simulink model "basic_cosimulation_c_1_sm_master"  (R2021b)
settings: Solver=ode4  StartTime=0.0  StopTime=inf  FixedStep=5e-05  RelTol=1e-3  EnableMultiTasking=on
PostLoadFcn:
  | %
  | % Script for validation of swtiching model design with it's respective
  | % average model.
  | %
  | % Here it is presented the design of the inverter to the 6 kW Fuel Cell
  | % model.
  | 
  | %%% Initialization %%%
  | 
  | 
  | % ------------------------------------- %
  | % ---------- Inverter Design ---------- %
  | % ------------------------------------- %
  | 
  | %%%% Nominal Parameters %%%%
  | 
  | Pnom = 50e3;                                        % Nominal Power
  | Vdc = 400;                                          % DC Voltage - Boost
  | m = 0.6;                                            % Modulation Index
  | Vnom_peak = m*Vdc/2;                                % Peak Voltage
  | Vnom_rms = Vnom_peak/sqrt(2);                       % Rms Voltage
  | FP_min = 0.9;                                       % For Reactive Power
  |                                                     % Compensation
  | Snom = Pnom/FP_min;                                 % Apparent Power
  | Irms = Pnom/(sqrt(3)*Vnom_rms);                     % Rms Curren
  | Inom_peak = Irms*sqrt(2);                           % Peak Current
  | Zbase = Vnom_peak/Inom_peak;                        % Base Impedance
  | f = 60;                                             % Nominal Frequency
  | wnom = 2*pi*60;                                     % Angular Frequency
  | 
  | % ------------------------- %
  | % Inverter LC Filter Design %
  | % ------------------------- %
  | 
  | fsw_inv = 96*60;                                    % Switching Frequency must be a multiple of the nominal frequency
  |                                                      % for proper operation of the Artemis Block
  | ripple_inv = 0.03;
  | L_inv = ((Vdc/2)-Vnom_peak)*(1/fsw_inv)/(ripple_inv*Inom_peak);
  | 
  | % - Capacitor
  | fres = 420;                                         % Filters Ressonant Frequency
  | 
  | Cf = 1/(4*L_inv*(pi^2)*(fres^2));                % Filter Capacitor
  | Rf = 1/(wnom*Cf*50);                                % Damping Resistor
  | 
  | % --- Sample Time --- %
  | 
  | Tsw = 0.00050;
  | Ts = Tsw/10;
  | 
  | % ---------------------- %
  | % Current Control Design %
  | % ---------------------- %
  | 
  | Ron = 0.001;                                        % IGBT Resistance
  | tau_i = 1e-3;                                       % Responde Time
  | kp_current = L_inv/tau_i;                           % PI Proportional Gain
  | ki_current = (Ron)/tau_i;                           % PI Integral Gain
  | 
  | decouple = (wnom*L_inv);                            % Decoupling Gain
InitFcn:
  | %
  | % Script for validation of swtiching model design with it's respective
  | % average model.
  | %
  | % Here it is presented the design of the inverter to the 6 kW Fuel Cell
  | % model.
  | 
  | %%% Initialization %%%
  | 
  | 
  | % ------------------------------------- %
  | % ---------- Inverter Design ---------- %
  | % ------------------------------------- %
  | 
  | %%%% Nominal Parameters %%%%
  | 
  | Pnom = 50e3;                                        % Nominal Power
  | Vdc = 400;                                          % DC Voltage - Boost
  | m = 0.6;                                            % Modulation Index
  | Vnom_peak = m*Vdc/2;                                % Peak Voltage
  | Vnom_rms = Vnom_peak/sqrt(2);                       % Rms Voltage
  | FP_min = 0.9;                                       % For Reactive Power
  |                                                     % Compensation
  | Snom = Pnom/FP_min;                                 % Apparent Power
  | Irms = Pnom/(sqrt(3)*Vnom_rms);                     % Rms Curren
  | Inom_peak = Irms*sqrt(2);                           % Peak Current
  | Zbase = Vnom_peak/Inom_peak;                        % Base Impedance
  | f = 60;                                             % Nominal Frequency
  | wnom = 2*pi*60;                                     % Angular Frequency
  | 
  | % ------------------------- %
  | % Inverter LC Filter Design %
  | % ------------------------- %
  | 
  | fsw_inv = 96*60;                                    % Switching Frequency must be a multiple of the nominal frequency
  |                                                      % for proper operation of the Artemis Block
  | ripple_inv = 0.03;
  | L_inv = ((Vdc/2)-Vnom_peak)*(1/fsw_inv)/(ripple_inv*Inom_peak);
  | 
  | % - Capacitor
  | fres = 420;                                         % Filters Ressonant Frequency
  | 
  | Cf = 1/(4*L_inv*(pi^2)*(fres^2));                % Filter Capacitor
  | Rf = 1/(wnom*Cf*50);                                % Damping Resistor
  | 
  | % --- Sample Time --- %
  | 
  | Tsw = 0.00050;
  | Ts = Tsw/10;
  | 
  | % ---------------------- %
  | % Current Control Design %
  | % ---------------------- %
  | 
  | Ron = 0.001;                                        % IGBT Resistance
  | tau_i = 1e-3;                                       % Responde Time
  | kp_current = L_inv/tau_i;                           % PI Proportional Gain
  | ki_current = (Ron)/tau_i;                           % PI Integral Gain
  | 
  | decouple = (wnom*L_inv);                            % Decoupling Gain
undefined symbols (not defined in the file or in its folder): D1, Delta, DiscIntNeverNeededParam, IP, j, ph, sps, UDP
libraries: powerlib x85, rtlab x16, spsCurrentMeasurementLib x11, powerlib_meascontrol x10, simulink x8, rteventslib x8, ssn_inverter_model x4, eePowerMeasurement x4, spsThreePhaseSeriesRLCBranchLib x4, spsVoltageMeasurementLib x4, opal_lib x3, spsUniversalBridgeLib x3
(part 2 of 5)

== system basic_cosimulation_c_1_sm_master/SM_Master/Circuit_ITM_Source_DP_AW ==
  Data_In : Inport
  AC Voltage Source : powerlib/Electrical Sources/AC Voltage Source  Commented=on  Amplitude=100  Phase=0  Frequency=60  SampleTime=0  Measurements=None  BusType=swing  Pref=10e3  Qref=0  Qmin=-inf  Qmax=+inf
  Amplitude : Step  Time=3  Before=220*sqrt(2/3)  After=220*sqrt(2/3)*0.8  SampleTime=Ts
  "Amplitude1 " : Step  Time=4  After=-220*sqrt(2/3)*0.2  SampleTime=Ts
  Constant : Constant  Commented=on  Value=5/60  SampleTime=Ts
  "Controllable Voltage Source " : Subsystem
  Controlled Current Source : powerlib/Electrical Sources/Controlled Current Source  Commented=on  Initialize=on  Source_Type=AC  Amplitude=0  Phase=0  Frequency=0  Measurements=None
  DP - > EMT : Subsystem
  DP --> EMT : Subsystem  Commented=on
  Demux1 : Demux  Outputs=3
  Digital Clock : DigitalClock  Commented=on  SampleTime=Ts
  Dynamic Phasor coeficientes extraction : Subsystem
  Dynamic Phasor coeficients extraction : Subsystem  Commented=on
  Freq : Step  Time=2.8  After=-2  SampleTime=Ts
  Freq Ref : Step  Time=2  Before=60  After=58  SampleTime=Ts
  GreaterThan : RelationalOperator  Commented=on  Operator=>  OutDataTypeStr=boolean  RndMeth=Simplest
  Ground1 : powerlib/Elements/Ground  Commented=on  LConnTagsString=a
  Mux : Mux  Inputs=3
  Mux1 : Mux  Inputs=3
  Phase Ref : Constant  Value=0  SampleTime=Ts
  Series RLC Branch : powerlib/Elements/Series RLC Branch  Commented=on  LConnTagsString=__new0  RConnTagsString=__new0  BranchType=R  Resistance=0.5  Inductance=1e-3  SetiL0=off  InitialCurrent=0  Capacitance=1e-6  Setx0=off  InitialVoltage=0  Measurements=None
  Subsystem : Subsystem  Commented=on
  Sum : Sum  Inputs=-+|
  Sum1 : Sum  Inputs=|+-
  Three-Phase Series RLC Branch1 : powerlib/Elements/Three-Phase Series RLC Branch  LConnTagsString=A|B|C  RConnTagsString=A|B|C  BranchType=R  Resistance=2  Inductance=1e-3  Capacitance=1e-6  Measurements=None
  Three-Phase V-I Measurement : powerlib/Measurements/Three-Phase V-I Measurement  VoltageMeasurement=phase-to-ground  SetLabelV=off  LabelV=Vabc  Vpu=off  VpuLL=off  CurrentMeasurement=yes  SetLabelI=off  LabelI=Iabc  Ipu=off  Pbase=100e6  Vbase=25e3  OutputType=Complex  PhasorSimulation=off  PSBequivalent=0
  Three-Phase Controlled Y-Connected Current Source : Subsystem
      settings: PortSchema="{\"entries\":[{\"content\":{\"sides\":[{\"content\":{\"connectorIds\":[\"LConn1\",\"LConn2\",\"LConn3\"]},\"type\":\"ConnectorPlacement.EquallySpacedRectSide\",\"uuid\":\"a8a67328-a09d-4495-b33c-aaf3ca0795cb\"},{\"content\":{\"connectorIds\":[\"In1\",\"In2\",\"In3\"],\"side\":\"RIGHT\"},\"type\":\"ConnectorPlacement.EquallySpacedRectSide\",\"uuid\":\"ca8d97e2-0dea-49aa-8cb7-235b4eace1f8\"},{\"content\":{\"connectorIds\":[],\"side\":\"TOP\"},\"type\":\"ConnectorPlacement.EquallySpacedRectSide\",\"uuid\":\"ab6aade9-1d27-4135-8ce1-c4358d4ecc87\"}]},\"type\":\"ConnectorPlacement.EquallySpacedConnector\",\"uuid\":\"205b5c38-55ea-4d68-a706-de660c21807c\"}],\"packageUris\":[\"http://schema.mathworks.com/mf0/Connector/19700101\"],\"version\":\"1.0\"}"
  Voltage Measurement : powerlib/Measurements/Voltage Measurement  Commented=on  PhasorSimulation=off  OutputType=Complex  PSBequivalent=0
  Vabc_Phasor_out : Outport
  I_injected : Outport  Port=2
  wires:
  DP --> EMT/1(I_injected) -> Controlled Current Source/1
  Voltage Measurement/1 -> Dynamic Phasor coeficients extraction/1(EMT Signal)
  Dynamic Phasor coeficients extraction/1(Mag) -> ?
  Dynamic Phasor coeficients extraction/2(Phase) -> ?
  Data_In/1 -> Demux1/1
  Three-Phase V-I Measurement/1 -> Dynamic Phasor coeficientes extraction/1(EMT_Signal)
  Dynamic Phasor coeficientes extraction/3(Phasor_C) -> Mux/3
  Dynamic Phasor coeficientes extraction/2(Phasor_B) -> Mux/2
  Dynamic Phasor coeficientes extraction/1(Phasor_A) -> Mux/1
  Mux/1 -> Vabc_Phasor_out/1
  Demux1/1 -> DP - > EMT/1(Phasor_A)
  Demux1/2 -> DP - > EMT/2(Phasor_B)
  Demux1/3 -> DP - > EMT/3(Phasor_C)
  DP - > EMT/2(Sinal_B) -> Mux1/2, Three-Phase Controlled Y-Connected Current Source/2(Ib)
  DP - > EMT/1(Sinal_A) -> Mux1/1, Three-Phase Controlled Y-Connected Current Source/1(Ia)
  DP - > EMT/3(Sinal_C) -> Mux1/3, Three-Phase Controlled Y-Connected Current Source/3(Ic)
  Mux1/1 -> I_injected/1
  Digital Clock/1 -> GreaterThan/1
  Constant/1 -> GreaterThan/2
  GreaterThan/1 -> ?
  Freq/1 -> Sum1/2
  Amplitude/1 -> Sum/2
  Sum/1 -> "Controllable Voltage Source "/1(Amplitude [V])
  Freq Ref/1 -> Sum1/1
  "Amplitude1 "/1 -> Sum/1
  Sum1/1 -> "Controllable Voltage Source "/3(Frequency [Hz])
  Phase Ref/1 -> "Controllable Voltage Source "/2(Phase [Deg])
  connections:
  AC Voltage Source/RConn1 -- Series RLC Branch/LConn1
  AC Voltage Source/LConn1 -- Controlled Current Source/RConn1 -- Voltage Measurement/LConn2 -- Ground1/LConn1
  Series RLC Branch/RConn1 -- Voltage Measurement/LConn1 -- Controlled Current Source/LConn1
  Three-Phase Series RLC Branch1/RConn2 -- Three-Phase V-I Measurement/LConn2
  Three-Phase V-I Measurement/LConn3 -- Three-Phase Series RLC Branch1/RConn3
  Three-Phase V-I Measurement/LConn1 -- Three-Phase Series RLC Branch1/RConn1
  Three-Phase Controlled Y-Connected Current Source/LConn1 -- Three-Phase V-I Measurement/RConn1
  Three-Phase V-I Measurement/RConn2 -- Three-Phase Controlled Y-Connected Current Source/LConn2
  Three-Phase V-I Measurement/RConn3 -- Three-Phase Controlled Y-Connected Current Source/LConn3
  "Controllable Voltage Source "/RConn1 -- Three-Phase Series RLC Branch1/LConn1
  Three-Phase Series RLC Branch1/LConn2 -- "Controllable Voltage Source "/RConn2
  Three-Phase Series RLC Branch1/LConn3 -- "Controllable Voltage Source "/RConn3

== system basic_cosimulation_c_1_sm_master/SM_Master/Circuit_ITM_Source_DP_SFA ==
  Data_In : Inport
  AC Voltage Source : powerlib/Electrical Sources/AC Voltage Source  Commented=on  Amplitude=100  Phase=0  Frequency=60  SampleTime=0  Measurements=None  BusType=swing  Pref=10e3  Qref=0  Qmin=-inf  Qmax=+inf
  Amplitude : Step  Time=3  Before=220*sqrt(2/3)  After=220*sqrt(2/3)*0.8  SampleTime=Ts
  "Amplitude1 " : Step  Time=4  After=-220*sqrt(2/3)*0.2  SampleTime=Ts
  "Controllable Voltage Source " : Subsystem
  Controlled Current Source : powerlib/Electrical Sources/Controlled Current Source  Commented=on  Initialize=on  Source_Type=AC  Amplitude=0  Phase=0  Frequency=0  Measurements=None
  DP --> EMT : Subsystem  Commented=on
  Dynamic Phasor coeficients extraction : Subsystem  Commented=on
  Freq : Step  Time=2.8  After=-2  SampleTime=Ts
  Freq Ref : Step  Time=2  Before=60  After=58  SampleTime=Ts
  Ground1 : powerlib/Elements/Ground  Commented=on  LConnTagsString=a
  Mux1 : Mux  Inputs=3
  Phase Ref : Constant  Value=0  SampleTime=Ts
  Phasor_to_Time_Domain_SFA : Subsystem  mask(Time domain from Dynamic Phasor){offset=60}
      mask prompts: offset "Frequency shift"
      mask help: This block extracts Time Domain Signals from the Dynamic Phasor by using the SFA method. It is usable only for three-phase signals
  Scope : Scope
  Series RLC Branch : powerlib/Elements/Series RLC Branch  Commented=on  LConnTagsString=__new0  RConnTagsString=__new0  BranchType=R  Resistance=0.5  Inductance=1e-3  SetiL0=off  InitialCurrent=0  Capacitance=1e-6  Setx0=off  InitialVoltage=0  Measurements=None
  Sum : Sum  Inputs=-+|
  Sum1 : Sum  Inputs=|+-
  Three-Phase Series RLC Branch1 : powerlib/Elements/Three-Phase Series RLC Branch  LConnTagsString=A|B|C  RConnTagsString=A|B|C  BranchType=R  Resistance=2  Inductance=1e-3  Capacitance=1e-6  Measurements=None
  Three-Phase V-I Measurement : powerlib/Measurements/Three-Phase V-I Measurement  VoltageMeasurement=phase-to-ground  SetLabelV=off  LabelV=Vabc  Vpu=off  VpuLL=off  CurrentMeasurement=yes  SetLabelI=off  LabelI=Iabc  Ipu=off  Pbase=100e6  Vbase=25e3  OutputType=Complex  PhasorSimulation=off  PSBequivalent=0
  Three-Phase Controlled Y-Connected Current Source : Subsystem
      settings: PortSchema="{\"entries\":[{\"content\":{\"sides\":[{\"content\":{\"connectorIds\":[\"LConn1\",\"LConn2\",\"LConn3\"]},\"type\":\"ConnectorPlacement.EquallySpacedRectSide\",\"uuid\":\"a8a67328-a09d-4495-b33c-aaf3ca0795cb\"},{\"content\":{\"connectorIds\":[\"In1\",\"In2\",\"In3\"],\"side\":\"RIGHT\"},\"type\":\"ConnectorPlacement.EquallySpacedRectSide\",\"uuid\":\"ca8d97e2-0dea-49aa-8cb7-235b4eace1f8\"},{\"content\":{\"connectorIds\":[],\"side\":\"TOP\"},\"type\":\"ConnectorPlacement.EquallySpacedRectSide\",\"uuid\":\"ab6aade9-1d27-4135-8ce1-c4358d4ecc87\"}]},\"type\":\"ConnectorPlacement.EquallySpacedConnector\",\"uuid\":\"205b5c38-55ea-4d68-a706-de660c21807c\"}],\"packageUris\":[\"http://schema.mathworks.com/mf0/Connector/19700101\"],\"version\":\"1.0\"}"
  Time_Domain_To_Phasor_SFA : Subsystem  mask(SFA){offset=60}
      mask prompts: offset "Frequency shift"
      mask help: This block extracts Dynamic Phasor by using the SFA method. It is usable only for three-phase signals
  Voltage Measurement : powerlib/Measurements/Voltage Measurement  Commented=on  PhasorSimulation=off  OutputType=Complex  PSBequivalent=0
  Vabc_Phasor_out : Outport
  I_injected : Outport  Port=2
  wires:
  DP --> EMT/1(I_injected) -> Controlled Current Source/1
  Voltage Measurement/1 -> Dynamic Phasor coeficients extraction/1(EMT Signal)
  Data_In/1 -> Phasor_to_Time_Domain_SFA/1(Dynamic_Phasor)
  Three-Phase V-I Measurement/1 -> Scope/1, Time_Domain_To_Phasor_SFA/1(EMT)
  Time_Domain_To_Phasor_SFA/1(Dynamic_Phasor) -> Vabc_Phasor_out/1
  Phasor_to_Time_Domain_SFA/1(A) -> Mux1/1, Three-Phase Controlled Y-Connected Current Source/1(Ia)
  Mux1/1 -> I_injected/1
  Phasor_to_Time_Domain_SFA/2(B) -> Mux1/2, Three-Phase Controlled Y-Connected Current Source/2(Ib)
  Phasor_to_Time_Domain_SFA/3(C) -> Mux1/3, Three-Phase Controlled Y-Connected Current Source/3(Ic)
  Phase Ref/1 -> "Controllable Voltage Source "/2(Phase [Deg])
  Amplitude/1 -> Sum/2
  Sum/1 -> "Controllable Voltage Source "/1(Amplitude [V])
  "Amplitude1 "/1 -> Sum/1
  Freq Ref/1 -> Sum1/1
  Sum1/1 -> "Controllable Voltage Source "/3(Frequency [Hz])
  Freq/1 -> Sum1/2
  connections:
  AC Voltage Source/RConn1 -- Series RLC Branch/LConn1
  AC Voltage Source/LConn1 -- Controlled Current Source/RConn1 -- Voltage Measurement/LConn2 -- Ground1/LConn1
  Series RLC Branch/RConn1 -- Voltage Measurement/LConn1 -- Controlled Current Source/LConn1
  Three-Phase Series RLC Branch1/RConn2 -- Three-Phase V-I Measurement/LConn2
  Three-Phase V-I Measurement/LConn3 -- Three-Phase Series RLC Branch1/RConn3
  Three-Phase V-I Measurement/LConn1 -- Three-Phase Series RLC Branch1/RConn1
  Three-Phase Controlled Y-Connected Current Source/LConn1 -- Three-Phase V-I Measurement/RConn1
  Three-Phase V-I Measurement/RConn2 -- Three-Phase Controlled Y-Connected Current Source/LConn2
  Three-Phase V-I Measurement/RConn3 -- Three-Phase Controlled Y-Connected Current Source/LConn3
  "Controllable Voltage Source "/RConn1 -- Three-Phase Series RLC Branch1/LConn1
  "Controllable Voltage Source "/RConn2 -- Three-Phase Series RLC Branch1/LConn2
  "Controllable Voltage Source "/RConn3 -- Three-Phase Series RLC Branch1/LConn3

== system basic_cosimulation_c_1_sm_master/SM_Master/OpComm ==
  Demux : Demux  Outputs="[1  2]"
  Receive : opal_lib/Communication/OpRecPar FromNT  Data_width=3  InitialConditions=[0;0;0]
  busStruct : Subsystem
  Out1 : Outport
  Out2 : Outport  Port=2
  wires:
  Demux/2 -> busStruct/2(In2)
  Demux/1 -> busStruct/1(In1)
  busStruct/2(Out2) -> Out2/1
  busStruct/1(Out1) -> Out1/1
  Receive/1 -> Demux/1

== system basic_cosimulation_c_1_sm_master/SM_Master/Original Circuit ==
  note: Inverter Measurements
  note: Model Control
  dblk : Inport
  PQ_ref : Inport  Port=2
  ARTEMiS SSN IVIC : ssn_inverter_model/ARTEMiS SSN IVIC  Arms=3  SnubberResistance=800  SnubberCapacitance=inf  Device=IGBT / Diodes  Ron=1e-3  Lon=0  ForwardVoltages=[0.001 0.001]  ForwardVoltage=0  GTOparameters=[ 10e-6 , 20e-6 ]  IGBTparameters=[ 1e-6 , 2e-6 ]*0  Measurements=None  Measurements_2=None  converterType=Rectifier
  Control : Subsystem
      settings: PortSchema="{\"entries\":[{\"content\":{\"sides\":[{\"content\":{\"connectorIds\":[\"In1\",\"In2\",\"In3\",\"In4\"]},\"type\":\"ConnectorPlacement.EquallySpacedRectSide\",\"uuid\":\"9324a1b5-9209-40a7-bba6-3b17f55cd5b4\"},{\"content\":{\"connectorIds\":[\"Out1\"],\"side\":\"RIGHT\"},\"type\":\"ConnectorPlacement.EquallySpacedRectSide\",\"uuid\":\"8b60fbd3-efee-4b93-84ca-13d5af533164\"},{\"content\":{\"connectorIds\":[],\"side\":\"TOP\"},\"type\":\"ConnectorPlacement.EquallySpacedRectSide\",\"uuid\":\"5aa46534-718a-472c-a25f-19e1867ae9eb\"},{\"content\":{\"connectorIds\":[\"Out2\"],\"side\":\"BOTTOM\"},\"type\":\"ConnectorPlacement.EquallySpacedRectSide\",\"uuid\":\"4a562f23-b1c9-4bd2-8d21-c9ff01dab3f7\"},{\"content\":{\"connectorIds\":[],\"side\":\"HIDDEN\"},\"type\":\"ConnectorPlacement.EquallySpacedRectSide\",\"uuid\":\"2bae700d-a0ed-419d-b89d-d5ddfcfc4dca\"}]},\"type\":\"ConnectorPlacement.EquallySpacedConnector\",\"uuid\":\"0ed67f90-7cb8-4c5b-bc99-423fd2f61638\"}],\"packageUris\":[\"http://schema.mathworks.com/mf0/Connector/R2020b\"],\"version\":\"1.0\"}"
  Current Measurement{,1..2,6} (4 alike) : spsCurrentMeasurementLib/Current Measurement  PhasorSimulation=off  OutputType=Complex  PSBequivalent=0
  DC Voltage Source : spsDCVoltageSourceLib/DC Voltage Source  Amplitude=Vdc  Measurements=None
  Delay : Delay  DelayLength=1
  Delay1 : Delay  DelayLength=1
  Delay2 : Delay  DelayLength=1
  Demux : Demux  Outputs=10
  Filter Capacitor : spsThreePhaseSeriesRLCBranchLib/Three-Phase Series RLC Branch  LConnTagsString=A|B|C  RConnTagsString=A|B|C  BranchType=RC  Resistance=Rf  Inductance=L_inv  Capacitance=Cf  Measurements=None
  Filter Inductor : spsThreePhaseSeriesRLCBranchLib/Three-Phase Series RLC Branch  LConnTagsString=A|B|C  RConnTagsString=A|B|C  BranchType=RL  Resistance=1e-3  Inductance=L_inv  Capacitance=1e-6  Measurements=None
  Iabc : Scope  NumInputPorts=3
  Icc_in : Scope
  Idq : Scope  NumInputPorts=2
  Mux : Mux  Inputs=2
  Mux1 : Mux  Inputs=3
  Mux2 : Mux  Inputs=6
  PWM : Subsystem  AncestorBlock=LafaeLib/PV System/PV System Detailed/VSC_Control/PWM
  Three-Phase Transformer (Two Windings) : spsThreePhaseTransformerTwoWindingsLib/Three-Phase Transformer (Two Windings)  Winding1Connection=Delta (D1)  Winding2Connection=Yg  CoreType=Three single-phase transformers  SetSaturation=off  Hysteresis=off  DataFile='hysteresis'  SetInitialFlux=off  Measurements=None  UNITS=pu  NominalPower=[ 80e3 , 60 ]  Winding1=[ Vnom_rms*sqrt(3) , 0.002 , 0.02 ]  Winding2=[440 , 0.002 , 0.02 ]  Rm=500  Lm=500  L0=0.5  Saturation=[ 0,0 ; 0.0024,1.2 ; 1.0,1.52 ]  InitialFluxes=[ 0.8 , -0.8 , 0.7 ]  BreakLoop=off  DiscreteSolver=Trapezoidal iterative  DataType=off  TransfoNumber=1
  Three-Phase Source : spsThreePhaseSourceLib/Three-Phase Source  InternalConnection=Yg  VoltagePhases=off  Voltage=440  PhaseAngle=0  Voltage_phases=[25e3 25e3 25e3]/sqrt(3)  PhaseAngles_phases=[0 -120 +120]  Frequency=60  NonIdealSource=on  SpecifyImpedance=off  Resistance=0.1e-3  Inductance=0.1e-3  ShortCircuitLevel=100e6  BaseVoltage=440  XRratio=7  BusType=swing  Pref=10e3  Qref=0  Prefabc=[10e3, 10e3, 10e3]  Qrefabc=[0, 0, 0]  Qmin=-inf  Qmax=inf
  Universal Bridge : spsUniversalBridgeLib/Universal Bridge  Commented=on  Arms=3  SnubberResistance=1e5  SnubberCapacitance=inf  Device=Average-model based VSC  Ron=1e-3  Lon=0  ForwardVoltages="[  0  0  ]"  ForwardVoltage=0  GTOparameters=[ 10e-6 , 20e-6 ]  IGBTparameters=[ 1e-6 , 2e-6 ]  Measurements=None  Measurements_2=None  converterType=Rectifier
  Vabc : Scope  NumInputPorts=3
  Vdq : Scope  NumInputPorts=2
  Voltage Measurement1 : spsVoltageMeasurementLib/Voltage Measurement  PhasorSimulation=off  OutputType=Complex  PSBequivalent=0
  Voltage Measurement2 : spsVoltageMeasurementLib/Voltage Measurement  PhasorSimulation=off  OutputType=Complex  PSBequivalent=0
  REF_V_I : Outport
  wires:
  dblk/1 -> [dblk]
  PQ_ref/1 -> [PQ_ref]
  Voltage Measurement1/1 -> Delay1/1
  Voltage Measurement2/1 -> Delay/1
  Current Measurement6/1 -> Icc_in/1
  Demux/1 -> Idq/1
  Control/1(Mabc) -> PWM/1(Uabc_ref)
  Delay1/1 -> [Vbc]
  Current Measurement/1 -> [ia]
  [dblk] -> Control/3(Deblock_inv)
  Demux/10 -> Mux2/6, Vabc/3
  Delay/1 -> [Vab]
  [Vab] -> Mux/1
  Delay2/1 -> Control/2(Iabc)
  [meas] -> Demux/1
  Demux/9 -> Mux2/5, Vabc/2
  Demux/2 -> Idq/2
  Demux/8 -> Vabc/1, Mux2/4
  Demux/3 -> Mux2/1, Iabc/1
  Demux/7 -> Vdq/2
  [ia] -> Mux1/1
  Control/2(Measures) -> [meas]
  [ib] -> Mux1/2
  [PQ_ref] -> Control/4(PQ_ref)
  Mux/1 -> Control/1(Vline)
  Demux/6 -> Vdq/1
  [Vbc] -> Mux/2
  Mux1/1 -> Delay2/1
  Demux/5 -> Iabc/3, Mux2/3
  Current Measurement2/1 -> [ic]
  Current Measurement1/1 -> [ib]
  [ic] -> Mux1/3
  PWM/1(Uref) -> ARTEMiS SSN IVIC/1
  Demux/4 -> Mux2/2, Iabc/2
  Mux2/1 -> REF_V_I/1
  connections:
  Filter Capacitor/LConn3 -- Voltage Measurement1/LConn2 -- Three-Phase Transformer (Two Windings)/LConn3 -- Current Measurement2/RConn1
  Filter Capacitor/RConn1 -- Filter Capacitor/RConn2 -- Filter Capacitor/RConn3
  Voltage Measurement1/LConn1 -- Three-Phase Transformer (Two Windings)/LConn2 -- Current Measurement1/RConn1 -- Filter Capacitor/LConn2 -- Voltage Measurement2/LConn2
  Three-Phase Transformer (Two Windings)/LConn1 -- Current Measurement/RConn1 -- Filter Capacitor/LConn1 -- Voltage Measurement2/LConn1
  Three-Phase Transformer (Two Windings)/RConn2 -- Three-Phase Source/RConn2
  DC Voltage Source/RConn1 -- Current Measurement6/LConn1
  Three-Phase Transformer (Two Windings)/RConn3 -- Three-Phase Source/RConn3
  Three-Phase Transformer (Two Windings)/RConn1 -- Three-Phase Source/RConn1
  ARTEMiS SSN IVIC/RConn2 -- DC Voltage Source/LConn1
  Current Measurement1/LConn1 -- Filter Inductor/RConn2
  Current Measurement6/RConn1 -- ARTEMiS SSN IVIC/RConn1
  ARTEMiS SSN IVIC/LConn2 -- Filter Inductor/LConn2
  ARTEMiS SSN IVIC/LConn1 -- Filter Inductor/LConn1
  Current Measurement2/LConn1 -- Filter Inductor/RConn3
  ARTEMiS SSN IVIC/LConn3 -- Filter Inductor/LConn3
  Current Measurement/LConn1 -- Filter Inductor/RConn1

== system basic_cosimulation_c_1_sm_master/SM_Master/Original_Circuit ==
  Amplitude : Step  Time=3  Before=220*sqrt(2/3)  After=220*sqrt(2/3)  SampleTime=Ts
  "Amplitude1 " : Step  Time=4  After=0  SampleTime=Ts
  "Controllable Voltage Source " : Subsystem
  Freq : Step  Time=2.8  After=0  SampleTime=Ts
  Freq Ref : Step  Time=2  Before=60  After=60  SampleTime=Ts
  Ground : powerlib/Elements/Ground  LConnTagsString=a
  Mux : Mux  Inputs=2
  Phase Ref : Constant  Value=0  SampleTime=Ts
  Sum : Sum  Inputs=-+|
  Sum1 : Sum  Inputs=|+-
  Three-Phase Series RLC Branch : powerlib/Elements/Three-Phase Series RLC Branch  LConnTagsString=A|B|C  RConnTagsString=A|B|C  BranchType=RL  Resistance=5  Inductance=1e-3  Capacitance=1e-6  Measurements=None
  Three-Phase Series RLC Branch1 : powerlib/Elements/Three-Phase Series RLC Branch  LConnTagsString=A|B|C  RConnTagsString=A|B|C  BranchType=R  Resistance=2  Inductance=1e-3  Capacitance=1e-6  Measurements=None
  Three-Phase V-I Measurement1 : powerlib/Measurements/Three-Phase V-I Measurement  VoltageMeasurement=phase-to-ground  SetLabelV=off  LabelV=Vabc  Vpu=off  VpuLL=off  CurrentMeasurement=yes  SetLabelI=off  LabelI=Iabc  Ipu=off  Pbase=100e6  Vbase=25e3  OutputType=Complex  PhasorSimulation=off  PSBequivalent=0
  Three-Phase Breaker : spsThreePhaseBreakerLib/Three-Phase Breaker  InitialState=open  SwitchA=on  SwitchB=on  SwitchC=on  SwitchTimes=[1]  External=off  BreakerResistance=0.001  SnubberResistance=1e6  SnubberCapacitance=inf  Measurements=None
  Vabc_Iabc_original : Outport
  wires:
  Three-Phase V-I Measurement1/1 -> Mux/1
  Three-Phase V-I Measurement1/2 -> Mux/2
  Mux/1 -> Vabc_Iabc_original/1
  Freq Ref/1 -> Sum1/1
  Sum/1 -> "Controllable Voltage Source "/1(Amplitude [V])
  Phase Ref/1 -> "Controllable Voltage Source "/2(Phase [Deg])
  Freq/1 -> Sum1/2
  Sum1/1 -> "Controllable Voltage Source "/3(Frequency [Hz])
  Amplitude/1 -> Sum/2
  "Amplitude1 "/1 -> Sum/1
  connections:
  Three-Phase V-I Measurement1/LConn2 -- Three-Phase Series RLC Branch1/RConn2
  Three-Phase V-I Measurement1/LConn1 -- Three-Phase Series RLC Branch1/RConn1
  Three-Phase V-I Measurement1/LConn3 -- Three-Phase Series RLC Branch1/RConn3
  Ground/LConn1 -- Three-Phase Series RLC Branch/RConn1 -- Three-Phase Series RLC Branch/RConn3 -- Three-Phase Series RLC Branch/RConn2
  "Controllable Voltage Source "/RConn2 -- Three-Phase Series RLC Branch1/LConn2
  "Controllable Voltage Source "/RConn1 -- Three-Phase Series RLC Branch1/LConn1
  "Controllable Voltage Source "/RConn3 -- Three-Phase Series RLC Branch1/LConn3
  Three-Phase Breaker/LConn1 -- Three-Phase V-I Measurement1/RConn1
  Three-Phase Breaker/LConn2 -- Three-Phase V-I Measurement1/RConn2
  Three-Phase Breaker/LConn3 -- Three-Phase V-I Measurement1/RConn3
  Three-Phase Breaker/RConn1 -- Three-Phase Series RLC Branch/LConn1
  Three-Phase Breaker/RConn2 -- Three-Phase Series RLC Branch/LConn2
  Three-Phase Breaker/RConn3 -- Three-Phase Series RLC Branch/LConn3

== system basic_cosimulation_c_1_sm_master/SM_Master/Saving RT Data ==
  group26 : Inport
  group27 : Inport  Port=2
  group28 : Inport  Port=3
  group29 : Inport  Port=4
  Bus to Vector{1..4} (4 alike) : BusToVector
  OpWriteFile26 : rtlab/DataLogging/OpWriteFile  Static_File=on  varname=data_send  Filename=data_send.mat  rtpath='./'  nrtpath='.\'  Acq_Group=26  file_size=(nls26+1)*8*(ld26/Ts)*1.5  write_offline=on  Sim_Mode=off  Nb_Samples=ld26/Ts  Buffer_size=(ld26/Ts)*8*(1+nls26)
      settings: SourceProductName=RT-LAB
  OpWriteFile27 : rtlab/DataLogging/OpWriteFile  Static_File=on  varname=data_recv  Filename=data_recv.mat  rtpath='./'  nrtpath='.\'  Acq_Group=27  file_size=(nls27+1)*8*(ld27/Ts)*1.5  write_offline=on  Sim_Mode=off  Nb_Samples=ld27/Ts  Buffer_size=(ld26/Ts)*8*(1+nls26)
      settings: SourceProductName=RT-LAB
  OpWriteFile28 : rtlab/DataLogging/OpWriteFile  Static_File=on  varname=I_injected  Filename=I_injected.mat  rtpath='./'  nrtpath='.\'  Acq_Group=28  file_size=(nls28+1)*8*(ld28/Ts)*1.5  write_offline=on  Sim_Mode=off  Nb_Samples=ld28/Ts  Buffer_size=(ld28/Ts)*8*(1+nls28)
      settings: SourceProductName=RT-LAB
  OpWriteFile29 : rtlab/DataLogging/OpWriteFile  Static_File=on  varname=Ref_V_I  Filename=Ref_V_I.mat  rtpath='./'  nrtpath='.\'  Acq_Group=29  file_size=(nls29+1)*8*(ld29/Ts)*1.5  write_offline=on  Sim_Mode=off  Nb_Samples=ld29/Ts  Buffer_size=(ld29/Ts)*8*(1+nls29)
      settings: SourceProductName=RT-LAB
  Terminator{1..8} (8 alike) : Terminator
  wires:
  OpWriteFile28/2 -> Terminator6/1
  OpWriteFile27/1 -> Terminator1/1
  OpWriteFile26/2 -> Terminator3/1
  OpWriteFile26/1 -> Terminator2/1
  OpWriteFile27/2 -> Terminator4/1
  OpWriteFile29/2 -> Terminator8/1
  OpWriteFile29/1 -> Terminator7/1
  OpWriteFile28/1 -> Terminator5/1
  group26/1 -> [group26]
  group27/1 -> [group27]
  group28/1 -> [group28]
  group29/1 -> [group29]
  [group27] -> Bus to Vector1/1
  Bus to Vector1/1 -> OpWriteFile27/1
  [group29] -> Bus to Vector2/1
  Bus to Vector2/1 -> OpWriteFile29/1
  [group26] -> Bus to Vector3/1
  Bus to Vector3/1 -> OpWriteFile26/1
  [group28] -> Bus to Vector4/1
  Bus to Vector4/1 -> OpWriteFile28/1

== system basic_cosimulation_c_1_sm_master/SM_Master/Saving RT Data1 ==
  group26 : Inport
  group27 : Inport  Port=2
  group28 : Inport  Port=3
  group29 : Inport  Port=4
  group30 : Inport  Port=5
  Bus to Vector{1..5} (5 alike) : BusToVector
  OpWriteFile26 : rtlab/DataLogging/OpWriteFile  Static_File=on  varname=data_send  Filename=data_send.mat  rtpath='./'  nrtpath='.\'  Acq_Group=26  file_size=(nls26+1)*8*(ld26/Ts)*1.5  write_offline=on  Sim_Mode=off  Nb_Samples=ld26/Ts  Buffer_size=(ld26/Ts)*8*(1+nls26)
      settings: SourceProductName=RT-LAB
  OpWriteFile27 : rtlab/DataLogging/OpWriteFile  Static_File=on  varname=data_recv  Filename=data_recv.mat  rtpath='./'  nrtpath='.\'  Acq_Group=27  file_size=(nls27+1)*8*(ld27/Ts)*1.5  write_offline=on  Sim_Mode=off  Nb_Samples=ld27/Ts  Buffer_size=(ld26/Ts)*8*(1+nls26)
      settings: SourceProductName=RT-LAB
  OpWriteFile28 : rtlab/DataLogging/OpWriteFile  Static_File=on  varname=V_injected  Filename=V_injected.mat  rtpath='./'  nrtpath='.\'  Acq_Group=28  file_size=(nls28+1)*8*(ld28/Ts)*1.5  write_offline=on  Sim_Mode=off  Nb_Samples=ld28/Ts  Buffer_size=(ld28/Ts)*8*(1+nls28)
      settings: SourceProductName=RT-LAB
  OpWriteFile29 : rtlab/DataLogging/OpWriteFile  Static_File=on  varname=Ref_V_I  Filename=Ref_V_I.mat  rtpath='./'  nrtpath='.\'  Acq_Group=29  file_size=(nls29+1)*8*(ld29/Ts)*1.5  write_offline=on  Sim_Mode=off  Nb_Samples=ld29/Ts  Buffer_size=(ld29/Ts)*8*(1+nls29)
      settings: SourceProductName=RT-LAB
  OpWriteFile30 : rtlab/DataLogging/OpWriteFile  Static_File=on  varname=PQ_ref  Filename=PQ_ref.mat  rtpath='./'  nrtpath='.\'  Acq_Group=30  file_size=(nls30+1)*8*(ld30/Ts)*1.5  write_offline=on  Sim_Mode=off  Nb_Samples=ld30/Ts  Buffer_size=(ld30/Ts)*8*(1+nls30)
      settings: SourceProductName=RT-LAB
  Terminator{1..10} (10 alike) : Terminator
  wires:
  OpWriteFile28/2 -> Terminator6/1
  OpWriteFile27/1 -> Terminator1/1
  OpWriteFile26/2 -> Terminator3/1
  OpWriteFile26/1 -> Terminator2/1
  OpWriteFile30/1 -> Terminator9/1
  OpWriteFile27/2 -> Terminator4/1
  OpWriteFile29/2 -> Terminator8/1
  OpWriteFile30/2 -> Terminator10/1
  OpWriteFile29/1 -> Terminator7/1
  OpWriteFile28/1 -> Terminator5/1
  group26/1 -> [group26]
  group27/1 -> [group27]
  group28/1 -> [group28]
  group29/1 -> [group29]
  group30/1 -> [group30]
  [group27] -> Bus to Vector1/1
  Bus to Vector1/1 -> OpWriteFile27/1
  [group29] -> Bus to Vector2/1
  Bus to Vector2/1 -> OpWriteFile29/1
  [group26] -> Bus to Vector3/1
  Bus to Vector3/1 -> OpWriteFile26/1
  [group28] -> Bus to Vector4/1
  Bus to Vector4/1 -> OpWriteFile28/1
  [group30] -> Bus to Vector5/1
  Bus to Vector5/1 -> OpWriteFile30/1

== system basic_cosimulation_c_1_sm_master/SM_Master/rtlab_send_subsystem ==
  Subsystem1 : Subsystem
  wires:
  [rtlab_send_1] -> Subsystem1/1(In1)
  [rtlab_send_2] -> Subsystem1/2(In2)
  [rtlab_send_3] -> Subsystem1/3(In3)
  [rtlab_send_4] -> Subsystem1/4(In4)
  [rtlab_send_5] -> Subsystem1/5(In5)

== system basic_cosimulation_c_1_sm_master/SM_Master/Circuit/Control ==
  note: Control
  note: Transformation
  note: 3 Wire and PLL
  Vline : Inport
  Iabc : Inport  Port=2
  Deblock_inv : Inport  Port=3
  PQ_ref : Inport  Port=4
  Current Control : Subsystem
      settings: PortSchema="{\"entries\":[{\"content\":{\"sides\":[{\"content\":{\"connectorIds\":[\"In1\",\"In2\",\"In3\",\"In4\"]},\"type\":\"ConnectorPlacement.EquallySpacedRectSide\",\"uuid\":\"45a39461-35bf-48e0-8374-0f28be422fe8\"},{\"content\":{\"connectorIds\":[\"Out1\"],\"side\":\"RIGHT\"},\"type\":\"ConnectorPlacement.EquallySpacedRectSide\",\"uuid\":\"af171a1a-fd9b-46cd-ac56-6e4044580109\"},{\"content\":{\"connectorIds\":[\"In5\"],\"side\":\"TOP\"},\"type\":\"ConnectorPlacement.EquallySpacedRectSide\",\"uuid\":\"ea73d2ad-6043-4637-ba6c-414a87cf6777\"},{\"content\":{\"connectorIds\":[],\"side\":\"HIDDEN\"},\"type\":\"ConnectorPlacement.EquallySpacedRectSide\",\"uuid\":\"ed240fd2-007a-443e-85e9-b2acea2870c2\"}]},\"type\":\"ConnectorPlacement.EquallySpacedConnector\",\"uuid\":\"aa40401b-6e13-445e-a9b0-89ce19fbc40c\"}],\"packageUris\":[\"http://schema.mathworks.com/mf0/Connector/R2020b\"],\"version\":\"1.0\"}"
  Currents : Scope  NumInputPorts=2
  Demux : Demux  Outputs=2
  Demux1 : Demux  Outputs=2
  Meas_3_Wire : Subsystem
  Modulation : Scope  Commented=on
  Mux1 : Mux  Inputs=5
  Mux2 : Mux  Inputs=2
  Park_Transformation : Subsystem
  Park_Transformation1 : Subsystem
  Power Control : Subsystem
      settings: PortSchema="{\"entries\":[{\"content\":{\"sides\":[{\"content\":{\"connectorIds\":[\"In1\"]},\"type\":\"ConnectorPlacement.EquallySpacedRectSide\",\"uuid\":\"974d39f2-3edd-4b06-9531-29f32c88933a\"},{\"content\":{\"connectorIds\":[\"Out1\"],\"side\":\"RIGHT\"},\"type\":\"ConnectorPlacement.EquallySpacedRectSide\",\"uuid\":\"24d62c8a-c61a-462a-84f0-1f0276c6dbaa\"},{\"content\":{\"connectorIds\":[],\"side\":\"TOP\"},\"type\":\"ConnectorPlacement.EquallySpacedRectSide\",\"uuid\":\"5ada6b1b-08a4-4e4d-9a20-cc19768e3a35\"},{\"content\":{\"connectorIds\":[\"In2\",\"In3\"],\"side\":\"BOTTOM\"},\"type\":\"ConnectorPlacement.EquallySpacedRectSide\",\"uuid\":\"aac35657-a4cf-4c82-a962-be637b231177\"},{\"content\":{\"connectorIds\":[],\"side\":\"HIDDEN\"},\"type\":\"ConnectorPlacement.EquallySpacedRectSide\",\"uuid\":\"6c2f95fb-9c8c-4eee-ad47-c57a643c3198\"}]},\"type\":\"ConnectorPlacement.EquallySpacedConnector\",\"uuid\":\"4f1b2c82-b884-470a-8be3-e486ca1ee764\"}],\"packageUris\":[\"http://schema.mathworks.com/mf0/Connector/R2020b\"],\"version\":\"1.0\"}"
  Power Measurement (Three-Phase) : eePowerMeasurement/Power Measurement (Three-Phase)  LabelModeActiveChoice=Discrete  F=60  K=[1]  Seq=Positive  Ts=Ts
      settings: SourceProductBaseCode=PS
  Product2 : Product
  SRF_PLL : Subsystem
  Saturation : Saturate  UpperLimit=1.1  LowerLimit=-1.1
  Terminator : Terminator
  Voltages : Scope  Commented=on  NumInputPorts=2
  Mabc : Outport
  Measures : Outport  Port=2
  Vabc : Outport  Port=3
  wires:
  SRF_PLL/1(Phase) -> [phase_pll]
  Park_Transformation/1(DQ) -> Currents/2, [Idq]
  [Vabc] -> SRF_PLL/1(Vabc)
  [Vabc] -> Voltages/1, Park_Transformation1/1(ABC)
  Park_Transformation1/1(DQ) -> Voltages/2, Demux1/1, [Vdq]
  [phase_pll] -> Park_Transformation1/2(Phase)
  Saturation/1 -> Mabc/1, Modulation/1
  [dblk] -> Product2/2
  Iabc/1 -> Park_Transformation/1(ABC), Currents/1, [Iabc]
  Meas_3_Wire/1(ABC) -> [Vabc]
  Product2/1 -> Saturation/1
  Vline/1 -> Demux/1
  Demux/1 -> Meas_3_Wire/1(AB)
  Demux/2 -> Meas_3_Wire/2(BC)
  Mux1/1 -> Measures/1
  [Vdq] -> Mux1/3
  [Iabc] -> Mux1/2
  [Vabc] -> Mux1/4, Vabc/1
  [Idq] -> Mux1/1
  Deblock_inv/1 -> [dblk], Current Control/1(Deblock)
  Current Control/1(modulation) -> Product2/1
  [Idq] -> Current Control/3(Idq)
  [Vdq] -> Current Control/4(Vdq)
  [phase_pll] -> Current Control/5(Phase)
  [phase_pll] -> Park_Transformation/2(Phase)
  Demux1/2 -> Terminator/1
  Demux1/1 -> [Vd]
  PQ_ref/1 -> Power Control/1(PQ_ref)
  [Vd] -> Power Control/2(Vd)
  [dblk] -> Power Control/3(Dblk)
  Power Control/1(Out1) -> Current Control/2(Idq_ref)
  [Vabc] -> Power Measurement (Three-Phase)/1
  [Iabc] -> Power Measurement (Three-Phase)/2
  Power Measurement (Three-Phase)/2 -> Mux2/2
  Power Measurement (Three-Phase)/1 -> Mux2/1
  Mux2/1 -> [pq_meas]
  [pq_meas] -> Mux1/5

== system basic_cosimulation_c_1_sm_master/SM_Master/Circuit/DP - > EMT ==
  Phasor_A : Inport
  Phasor_B : Inport  Port=2
  Phasor_C : Inport  Port=3
  Demux : Demux  Outputs=2
  Demux1 : Demux  Outputs=2
  Demux2 : Demux  Outputs=2
  Subsystem : Subsystem
  Subsystem1 : Subsystem
  Subsystem2 : Subsystem
  Sinal_A : Outport
  Sinal_B : Outport  Port=2
  Sinal_C : Outport  Port=3
  wires:
  Subsystem2/1(Out1) -> Sinal_C/1
  Subsystem1/1(Out1) -> Sinal_B/1
  Subsystem/1(Out1) -> Sinal_A/1
  Demux/1 -> Subsystem/1(In1)
  Demux/2 -> Subsystem/2(Input)
  Demux1/1 -> Subsystem1/1(In1)
  Demux1/2 -> Subsystem1/2(Input1)
  Demux2/1 -> Subsystem2/1(In1)
  Demux2/2 -> Subsystem2/2(Input2)
  Phasor_A/1 -> Demux/1
  Phasor_B/1 -> Demux1/1
  Phasor_C/1 -> Demux2/1

== system basic_cosimulation_c_1_sm_master/SM_Master/Circuit/Dynamic Phasor coeficientes extraction ==
  EMT_Signal : Inport
  Demux : Demux  Outputs=3
  Fourier_A : powerlib_meascontrol/Measurements/Fourier  Freq=60  n=1  InInit=[1,0]  Ts=Ts
  Fourier_B : powerlib_meascontrol/Measurements/Fourier  Freq=60  n=1  InInit=[1,-120 ]  Ts=Ts
  Fourier_C : powerlib_meascontrol/Measurements/Fourier  Freq=60  n=1  InInit=[1,+120 ]  Ts=Ts
  Mux : Mux  Inputs=2
  Mux1 : Mux  Inputs=2
  Mux2 : Mux  Inputs=2
  deg->rad : Gain  Gain=pi/180  SaturateOnIntegerOverflow=on  OutDataTypeStr=Inherit: Same as input  ParamDataTypeStr=Inherit: Same as input
  deg->rad1 : Gain  Gain=pi/180  SaturateOnIntegerOverflow=on  OutDataTypeStr=Inherit: Same as input  ParamDataTypeStr=Inherit: Same as input
  deg->rad2 : Gain  Gain=pi/180  SaturateOnIntegerOverflow=on  OutDataTypeStr=Inherit: Same as input  ParamDataTypeStr=Inherit: Same as input
  Phasor_A : Outport
  Phasor_B : Outport  Port=2
  Phasor_C : Outport  Port=3
  wires:
  Demux/2 -> Fourier_B/1
  deg->rad1/1 -> Mux2/2
  Demux/3 -> Fourier_C/1
  Demux/1 -> Fourier_A/1
  Fourier_C/1 -> Mux1/1
  EMT_Signal/1 -> Demux/1
  Fourier_B/2 -> deg->rad1/1
  deg->rad2/1 -> Mux1/2
  Fourier_A/2 -> deg->rad/1
  Fourier_C/2 -> deg->rad2/1
  Fourier_A/1 -> Mux/1
  deg->rad/1 -> Mux/2
  Fourier_B/1 -> Mux2/1
  Mux/1 -> Phasor_A/1
  Mux2/1 -> Phasor_B/1
  Mux1/1 -> Phasor_C/1

== system basic_cosimulation_c_1_sm_master/SM_Master/Circuit/PWM ==
  Uabc_ref : Inport
  Constant10 : Constant  Value=2
  Constant11 : Constant  Value=fsw_inv
  Constant9 : Constant
  Demux8 : Demux  Outputs=3
  Divide7 : Product  Inputs=*/
  Divide8 : Product  Inputs=*/
  Divide9 : Product  Inputs=*/
  Mux11 : Mux  Inputs=3
  Mux12 : Mux  Inputs=2
  RTE Conversion1 : rteventslib/Signal Attributes/RTE Conversion  inputdatatype=RTE Boolean  outputdatatype=Double  compensation=Enabled  nbMaxEvents=4  sampleTime=Ts
  RTE SPWM1 : rteventslib/Sources/RTE SPWM  NumberPhases=3-ph  CenterAlignmentMode=On  MaxFreq=inf  MinFreq=0  EnablingPort=off  ComplementaryMode=on  SpaceVector=off  RiseTimeDelay=0  MaxEvents=4  SampleTime=Ts
  Scope : Scope
  Scope8 : Scope
  Selector1 : Selector  InputPortWidth=6  IndexOptions=Index vector (dialog)  Indices=[1 4 2 5 3 6]  OutputSizes=1
  Sum16 : Sum  Inputs=|++
  Sum17 : Sum  Inputs=|++
  Sum18 : Sum  Inputs=|++
  Uref : Outport  VectorParamsAs1DForOutWhenUnconnected=off
  wires:
  Uabc_ref/1 -> Demux8/1, Scope/1
  RTE SPWM1/1 -> Mux12/1
  Constant9/1 -> Sum18/2, Sum17/2, Sum16/2
  Selector1/1 -> Uref/1
  Constant11/1 -> RTE SPWM1/1
  Sum16/1 -> Divide7/1
  Constant10/1 -> Divide9/2, Divide8/2, Divide7/2
  Sum17/1 -> Divide8/1
  Divide9/1 -> Mux11/3
  RTE SPWM1/2 -> Mux12/2
  Demux8/2 -> Sum17/1
  Divide8/1 -> Mux11/2
  Sum18/1 -> Divide9/1
  Mux11/1 -> RTE SPWM1/2, Scope8/1
  Divide7/1 -> Mux11/1
  Demux8/1 -> Sum16/1
  Demux8/3 -> Sum18/1
  Mux12/1 -> RTE Conversion1/1
  RTE Conversion1/1 -> Selector1/1

== system basic_cosimulation_c_1_sm_master/SM_Master/Circuit/Three-Phase Controlled Y-Connected Voltage Source  ==
  Va : Inport
  Vb : Inport  Port=2
  Vc : Inport  Port=3
  Controlled Voltage Source : powerlib/Electrical Sources/Controlled Voltage Source  Initialize=off  Source_Type=AC  Amplitude=0  Phase=0  Frequency=0  Measurements=None
  Controlled Voltage Source1 : powerlib/Electrical Sources/Controlled Voltage Source  Initialize=off  Source_Type=AC  Amplitude=0  Phase=0  Frequency=0  Measurements=None
  Controlled Voltage Source2 : powerlib/Electrical Sources/Controlled Voltage Source  Initialize=off  Source_Type=AC  Amplitude=0  Phase=0  Frequency=0  Measurements=None
  Ground : powerlib/Elements/Ground  LConnTagsString=a
  + : PMIOPort  Side=Right
  +1 : PMIOPort  Port=2  Side=Right
  +2 : PMIOPort  Port=3  Side=Right
  wires:
  Vb/1 -> Controlled Voltage Source1/1
  Va/1 -> Controlled Voltage Source/1
  Vc/1 -> Controlled Voltage Source2/1
  connections:
  Controlled Voltage Source/RConn1 -- +/RConn1
  Controlled Voltage Source1/RConn1 -- +1/RConn1
  Controlled Voltage Source2/RConn1 -- +2/RConn1
  Controlled Voltage Source2/LConn1 -- Controlled Voltage Source/LConn1 -- Controlled Voltage Source1/LConn1 -- Ground/LConn1

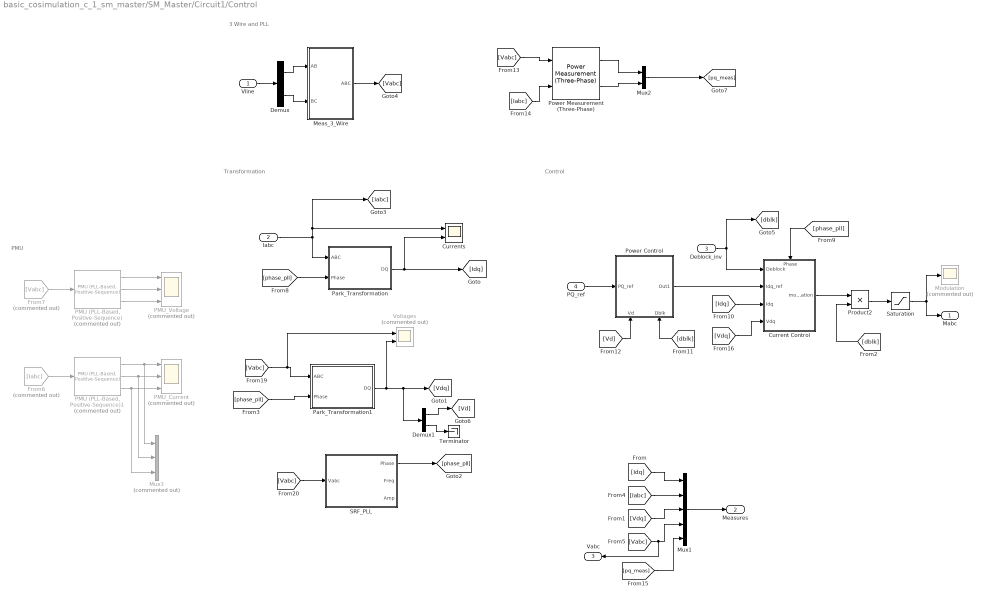
== system basic_cosimulation_c_1_sm_master/SM_Master/Circuit1/Control ==
  note: PMU
  note: Control
  note: Transformation
  note: 3 Wire and PLL
  Vline : Inport
  Iabc : Inport  Port=2
  Deblock_inv : Inport  Port=3
  PQ_ref : Inport  Port=4
  Current Control : Subsystem
      settings: PortSchema="{\"entries\":[{\"content\":{\"sides\":[{\"content\":{\"connectorIds\":[\"In1\",\"In2\",\"In3\",\"In4\"]},\"type\":\"ConnectorPlacement.EquallySpacedRectSide\",\"uuid\":\"45a39461-35bf-48e0-8374-0f28be422fe8\"},{\"content\":{\"connectorIds\":[\"Out1\"],\"side\":\"RIGHT\"},\"type\":\"ConnectorPlacement.EquallySpacedRectSide\",\"uuid\":\"af171a1a-fd9b-46cd-ac56-6e4044580109\"},{\"content\":{\"connectorIds\":[\"In5\"],\"side\":\"TOP\"},\"type\":\"ConnectorPlacement.EquallySpacedRectSide\",\"uuid\":\"ea73d2ad-6043-4637-ba6c-414a87cf6777\"},{\"content\":{\"connectorIds\":[],\"side\":\"HIDDEN\"},\"type\":\"ConnectorPlacement.EquallySpacedRectSide\",\"uuid\":\"ed240fd2-007a-443e-85e9-b2acea2870c2\"}]},\"type\":\"ConnectorPlacement.EquallySpacedConnector\",\"uuid\":\"aa40401b-6e13-445e-a9b0-89ce19fbc40c\"}],\"packageUris\":[\"http://schema.mathworks.com/mf0/Connector/R2020b\"],\"version\":\"1.0\"}"
  Currents : Scope  NumInputPorts=2
  Demux : Demux  Outputs=2
  Demux1 : Demux  Outputs=2
  From6 : From  Commented=on  GotoTag=Iabc
  From7 : From  Commented=on  GotoTag=Vabc
  Meas_3_Wire : Subsystem
  Modulation : Scope  Commented=on
  Mux1 : Mux  Inputs=5
  Mux2 : Mux  Inputs=2
  Mux3 : Mux  Commented=on  Inputs=3
  "PMU (PLL-Based, Positive-Sequence)" : spsPMUPLLBasedPositiveSequenceLib/PMU (PLL-Based, Positive-Sequence)  Commented=on  nominalFrequency=60  samplingRate=48  reportingFactor=1
      settings: SourceProductBaseCode=PS
  "PMU (PLL-Based, Positive-Sequence)1" : spsPMUPLLBasedPositiveSequenceLib/PMU (PLL-Based, Positive-Sequence)  Commented=on  nominalFrequency=60  samplingRate=48  reportingFactor=1
      settings: SourceProductBaseCode=PS
  PMU_Current : Scope  Commented=on  NumInputPorts=3
  PMU_Voltage : Scope  Commented=on  NumInputPorts=3
  Park_Transformation : Subsystem
  Park_Transformation1 : Subsystem
  Power Control : Subsystem
      settings: PortSchema="{\"entries\":[{\"content\":{\"sides\":[{\"content\":{\"connectorIds\":[\"In1\"]},\"type\":\"ConnectorPlacement.EquallySpacedRectSide\",\"uuid\":\"974d39f2-3edd-4b06-9531-29f32c88933a\"},{\"content\":{\"connectorIds\":[\"Out1\"],\"side\":\"RIGHT\"},\"type\":\"ConnectorPlacement.EquallySpacedRectSide\",\"uuid\":\"24d62c8a-c61a-462a-84f0-1f0276c6dbaa\"},{\"content\":{\"connectorIds\":[],\"side\":\"TOP\"},\"type\":\"ConnectorPlacement.EquallySpacedRectSide\",\"uuid\":\"5ada6b1b-08a4-4e4d-9a20-cc19768e3a35\"},{\"content\":{\"connectorIds\":[\"In2\",\"In3\"],\"side\":\"BOTTOM\"},\"type\":\"ConnectorPlacement.EquallySpacedRectSide\",\"uuid\":\"aac35657-a4cf-4c82-a962-be637b231177\"},{\"content\":{\"connectorIds\":[],\"side\":\"HIDDEN\"},\"type\":\"ConnectorPlacement.EquallySpacedRectSide\",\"uuid\":\"6c2f95fb-9c8c-4eee-ad47-c57a643c3198\"}]},\"type\":\"ConnectorPlacement.EquallySpacedConnector\",\"uuid\":\"4f1b2c82-b884-470a-8be3-e486ca1ee764\"}],\"packageUris\":[\"http://schema.mathworks.com/mf0/Connector/R2020b\"],\"version\":\"1.0\"}"
  Power Measurement (Three-Phase) : eePowerMeasurement/Power Measurement (Three-Phase)  LabelModeActiveChoice=Discrete  F=60  K=[1]  Seq=Positive  Ts=Ts
      settings: SourceProductBaseCode=PS
  Product2 : Product
  SRF_PLL : Subsystem
  Saturation : Saturate  UpperLimit=1.1  LowerLimit=-1.1
  Terminator : Terminator
  Voltages : Scope  Commented=on  NumInputPorts=2
  Mabc : Outport
  Measures : Outport  Port=2
  Vabc : Outport  Port=3
  wires:
  SRF_PLL/1(Phase) -> [phase_pll]
  Park_Transformation/1(DQ) -> Currents/2, [Idq]
  [Vabc] -> SRF_PLL/1(Vabc)
  [Vabc] -> Voltages/1, Park_Transformation1/1(ABC)
  Park_Transformation1/1(DQ) -> Voltages/2, Demux1/1, [Vdq]
  [phase_pll] -> Park_Transformation1/2(Phase)
  Saturation/1 -> Mabc/1, Modulation/1
  [dblk] -> Product2/2
  Iabc/1 -> Park_Transformation/1(ABC), Currents/1, [Iabc]
  Meas_3_Wire/1(ABC) -> [Vabc]
  Product2/1 -> Saturation/1
  Vline/1 -> Demux/1
  Demux/1 -> Meas_3_Wire/1(AB)
  Demux/2 -> Meas_3_Wire/2(BC)
  Mux1/1 -> Measures/1
  [Vdq] -> Mux1/3
  [Iabc] -> Mux1/2
  [Vabc] -> Mux1/4, Vabc/1
  [Idq] -> Mux1/1
  From7/1 -> "PMU (PLL-Based, Positive-Sequence)"/1
  From6/1 -> "PMU (PLL-Based, Positive-Sequence)1"/1
  "PMU (PLL-Based, Positive-Sequence)"/1 -> PMU_Voltage/1
  "PMU (PLL-Based, Positive-Sequence)"/2 -> PMU_Voltage/2
  "PMU (PLL-Based, Positive-Sequence)"/3 -> PMU_Voltage/3
  "PMU (PLL-Based, Positive-Sequence)1"/1 -> Mux3/1, PMU_Current/1
  "PMU (PLL-Based, Positive-Sequence)1"/2 -> Mux3/2, PMU_Current/2
  "PMU (PLL-Based, Positive-Sequence)1"/3 -> Mux3/3, PMU_Current/3
  Deblock_inv/1 -> [dblk], Current Control/1(Deblock)
  Current Control/1(modulation) -> Product2/1
  [Idq] -> Current Control/3(Idq)
  [Vdq] -> Current Control/4(Vdq)
  [phase_pll] -> Current Control/5(Phase)
  [phase_pll] -> Park_Transformation/2(Phase)
  Demux1/2 -> Terminator/1
  Demux1/1 -> [Vd]
  PQ_ref/1 -> Power Control/1(PQ_ref)
  [Vd] -> Power Control/2(Vd)
  [dblk] -> Power Control/3(Dblk)
  Power Control/1(Out1) -> Current Control/2(Idq_ref)
  [Vabc] -> Power Measurement (Three-Phase)/1
  [Iabc] -> Power Measurement (Three-Phase)/2
  Power Measurement (Three-Phase)/2 -> Mux2/2
  Power Measurement (Three-Phase)/1 -> Mux2/1
  Mux2/1 -> [pq_meas]
  [pq_meas] -> Mux1/5

== system basic_cosimulation_c_1_sm_master/SM_Master/Circuit1/PWM ==
  Uabc_ref : Inport
  Constant10 : Constant  Value=2
  Constant11 : Constant  Value=fsw_inv
  Constant9 : Constant
  Demux8 : Demux  Outputs=3
  Divide7 : Product  Inputs=*/
  Divide8 : Product  Inputs=*/
  Divide9 : Product  Inputs=*/
  Mux11 : Mux  Inputs=3
  Mux12 : Mux  Inputs=2
  RTE Conversion1 : rteventslib/Signal Attributes/RTE Conversion  inputdatatype=RTE Boolean  outputdatatype=Double  compensation=Enabled  nbMaxEvents=4  sampleTime=Ts
  RTE SPWM1 : rteventslib/Sources/RTE SPWM  NumberPhases=3-ph  CenterAlignmentMode=On  MaxFreq=inf  MinFreq=0  EnablingPort=off  ComplementaryMode=on  SpaceVector=off  RiseTimeDelay=0  MaxEvents=4  SampleTime=Ts
  Scope : Scope
  Scope8 : Scope
  Selector1 : Selector  InputPortWidth=6  IndexOptions=Index vector (dialog)  Indices=[1 4 2 5 3 6]  OutputSizes=1
  Sum16 : Sum  Inputs=|++
  Sum17 : Sum  Inputs=|++
  Sum18 : Sum  Inputs=|++
  Uref : Outport  VectorParamsAs1DForOutWhenUnconnected=off
  wires:
  Uabc_ref/1 -> Demux8/1, Scope/1
  RTE SPWM1/1 -> Mux12/1
  Constant9/1 -> Sum18/2, Sum17/2, Sum16/2
  Selector1/1 -> Uref/1
  Constant11/1 -> RTE SPWM1/1
  Sum16/1 -> Divide7/1
  Constant10/1 -> Divide9/2, Divide8/2, Divide7/2
  Sum17/1 -> Divide8/1
  Divide9/1 -> Mux11/3
  RTE SPWM1/2 -> Mux12/2
  Demux8/2 -> Sum17/1
  Divide8/1 -> Mux11/2
  Sum18/1 -> Divide9/1
  Mux11/1 -> RTE SPWM1/2, Scope8/1
  Divide7/1 -> Mux11/1
  Demux8/1 -> Sum16/1
  Demux8/3 -> Sum18/1
  Mux12/1 -> RTE Conversion1/1
  RTE Conversion1/1 -> Selector1/1
